simulink model "controllo_leggelin_e_quad"  (R2019b)
settings: Solver=FixedStepAuto  StartTime=0.0  StopTime=t_tot  FixedStep=dt  RelTol=1e-3
values from neighbouring files (symbols this model uses):
  A = [0 0 1 0; 0 0 0 1; 0 a_32  0 a_34; a_41 a_42 0 a_44]    [QuarterCarModel.m]
  B = [0; 0; 0; -kt/mu]    [QuarterCarModel.m]
  C = [0 -k/ms 0 -c_min/ms]    [QuarterCarModel.m]
  c_min = 800    [QuarterCarModel.m]
  er = 0.7    [QuarterCarModel.m]
  f_max = 3000    [QuarterCarModel.m]
  k = 27000    [QuarterCarModel.m]
  k0 = 38000    [QuarterCarModel.m]
  k_tilde = best_Ktilde    [QuarterCarModel.m]    (also in fun_lin.m = [x.k1 x.k2 x.k3 x.k4]; fun_lin_e_quad.m = [x.k1 0 x.k3 x.k4])
  kt = 300000    [QuarterCarModel.m]
  ms = 450    [QuarterCarModel.m]
  mu = 70    [QuarterCarModel.m]
  Px = best_elementsP    [QuarterCarModel.m]    (also in fun_lin_e_quad.m = [0 0 x.p13  x.p14; 0 0 0 0; x.p13 0 0  x.p34;  x.p14 0  x.p3; fun_quad.m = [x.p11 0 x.p13  x.p14; 0 0 0 0; x.p13 0 x.p33  x.p34;  x.p14)
  wr = 2*pi*v/lc    (= 7.85398163397)    [QuarterCarModel.m]
libraries: simulink x2
settings Model: Creator=Elia  LastModifiedBy=Elia

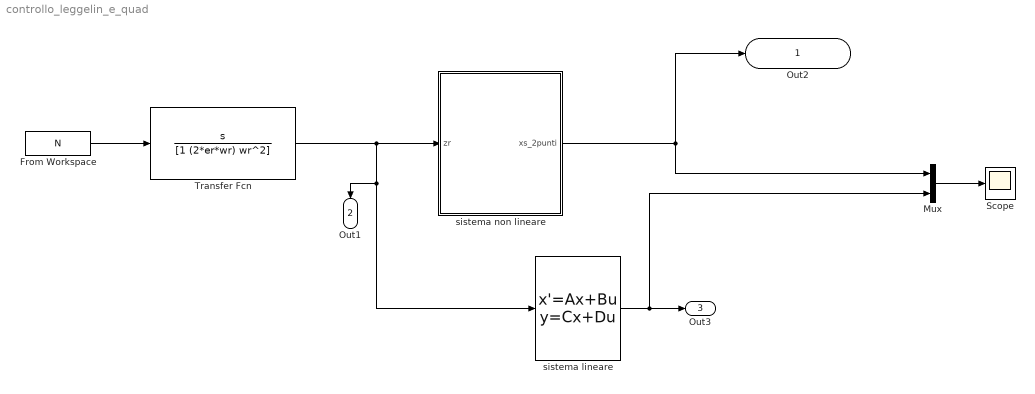
== system controllo_leggelin_e_quad ==
  From Workspace : FromWorkspace  VariableName=N  SampleTime=0
  Mux : Mux  Inputs=2
  Scope : Scope
  Transfer Fcn : TransferFcn  Numerator=[1 0]  Denominator=[1 (2*er*wr) wr^2]
  sistema lineare : StateSpace  A=A  B=B  C=C  D=0  InitialCondition=0
  sistema non lineare : Subsystem
  Out2 : Outport  SignalName=xs_2punti
  Out1 : Outport  Port=2  SignalName=zr
  Out3 : Outport  Port=3  SignalName=xs_2punti_lineare
  wires:
  sistema non lineare/1(xs_2punti) -> Mux/1, Out2/1
  From Workspace/1 -> Transfer Fcn/1
  Transfer Fcn/1 -> sistema non lineare/1(zr), sistema lineare/1, Out1/1
  sistema lineare/1 -> Mux/2, Out3/1
  Mux/1 -> Scope/1

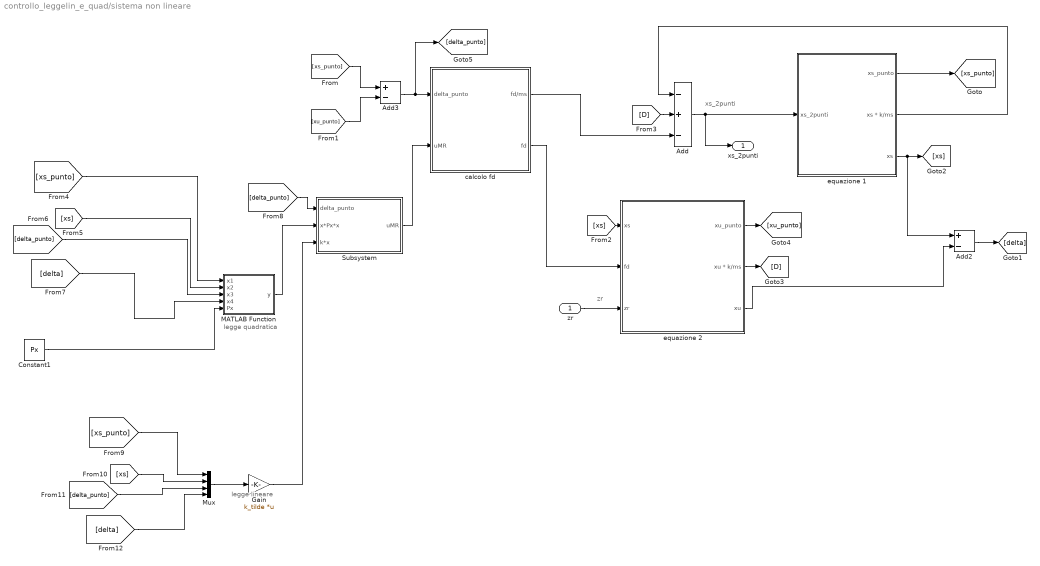
== system controllo_leggelin_e_quad/sistema non lineare ==
  note: legge quadratica
  note: xs_2punti
  note: zr
  note: legge lineare
  zr : Inport
  Add : Sum  Inputs=-+-
  Add2 : Sum  Inputs=+-
  Add3 : Sum  Inputs=+-
  Constant1 : Constant  Value=Px
  Gain : Gain  Gain=k_tilde  Multiplication=Matrix(K*u)
  MATLAB Function : MATLAB Function  TreatAsAtomicUnit=on
  Mux : Mux
  Subsystem : Subsystem
  calcolo fd : Subsystem
  equazione 1 : Subsystem
  equazione 2 : Subsystem
  xs_2punti : Outport
  wires:
  calcolo fd/2(fd) -> equazione 2/2(fd)
  equazione 1/3(xs) -> Add2/1, [xs]
  Add/1 -> xs_2punti/1, equazione 1/1(xs_2punti)
  equazione 1/1(xs_punto) -> [xs_punto]
  calcolo fd/1(fd/ms) -> Add/3
  [xs] -> equazione 2/1(xs)
  [D] -> Add/2
  equazione 1/2("xs * k/ms ") -> Add/1
  equazione 2/2("xu * k/ms ") -> [D]
  zr/1 -> equazione 2/3(zr)
  equazione 2/3(xu) -> Add2/2
  equazione 2/1(xu_punto) -> [xu_punto]
  [xu_punto] -> Add3/2
  [xs_punto] -> Add3/1
  Add3/1 -> [delta_punto], calcolo fd/1("delta_punto ")
  Add2/1 -> [delta]
  [delta_punto] -> Subsystem/1(delta_punto)
  MATLAB Function/1(y) -> Subsystem/2(x*Px*x)
  Constant1/1 -> MATLAB Function/5(Px)
  [xs_punto] -> MATLAB Function/1(x1)
  [xs] -> MATLAB Function/2(x2)
  [delta_punto] -> MATLAB Function/3(x3)
  [delta] -> MATLAB Function/4(x4)
  Subsystem/1(uMR) -> calcolo fd/2(uMR)
  [delta_punto] -> Mux/3
  [delta] -> Mux/4
  Mux/1 -> Gain/1
  [xs] -> Mux/2
  [xs_punto] -> Mux/1
  Gain/1 -> Subsystem/3(k*x)

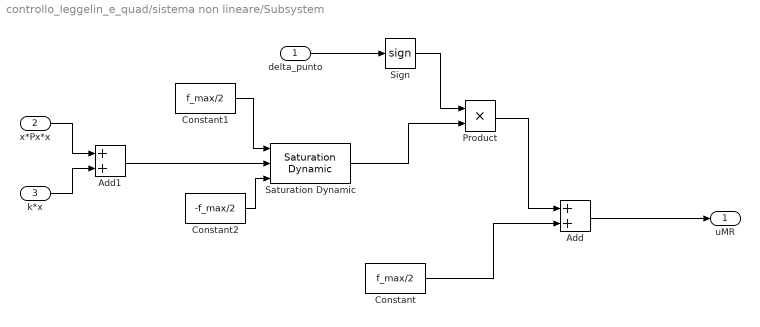
== system controllo_leggelin_e_quad/sistema non lineare/Subsystem ==
  delta_punto : Inport
  x*Px*x : Inport  Port=2
  k*x : Inport  Port=3
  Add : Sum
  Add1 : Sum
  Constant : Constant  Value=f_max/2
  Constant1 : Constant  Value=f_max/2
  Constant2 : Constant  Value=-f_max/2
  Product : Product
  Saturation Dynamic : simulink/Discontinuities/Saturation Dynamic  OutMin=[]  OutMax=[]  OutDataTypeStr=Inherit: Same as second input  OutDataType=fixdt(1, 16)  OutScaling=2^-10  DoSatur=off
  Sign : Signum
  uMR : Outport
  wires:
  Constant/1 -> Add/2
  Add/1 -> uMR/1
  delta_punto/1 -> Sign/1
  Saturation Dynamic/1 -> Product/2
  Sign/1 -> Product/1
  Product/1 -> Add/1
  Constant1/1 -> Saturation Dynamic/1
  Constant2/1 -> Saturation Dynamic/3
  x*Px*x/1 -> Add1/1
  k*x/1 -> Add1/2
  Add1/1 -> Saturation Dynamic/2

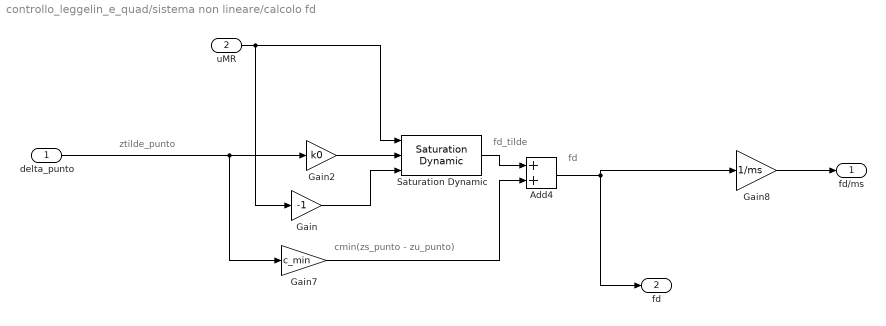
== system controllo_leggelin_e_quad/sistema non lineare/calcolo fd ==
  note: ztilde_punto
  note: cmin(zs_punto - zu_punto)
  note: fd
  note: fd_tilde
  "delta_punto " : Inport
  uMR : Inport  Port=2
  Add4 : Sum
  Gain : Gain  Gain=-1
  Gain2 : Gain  Gain=k0
  Gain7 : Gain  Gain=c_min
  Gain8 : Gain  Gain=1/ms
  Saturation Dynamic : simulink/Discontinuities/Saturation Dynamic  OutMin=[]  OutMax=[]  OutDataTypeStr=Inherit: Same as second input  OutDataType=fixdt(1, 16)  OutScaling=2^-10  DoSatur=off
  fd/ms : Outport
  fd : Outport  Port=2
  wires:
  "delta_punto "/1 -> Gain2/1, Gain7/1
  Gain2/1 -> Saturation Dynamic/2
  Add4/1 -> Gain8/1, fd/1
  Gain8/1 -> fd/ms/1
  Gain7/1 -> Add4/2
  Saturation Dynamic/1 -> Add4/1
  uMR/1 -> Gain/1, Saturation Dynamic/1
  Gain/1 -> Saturation Dynamic/3

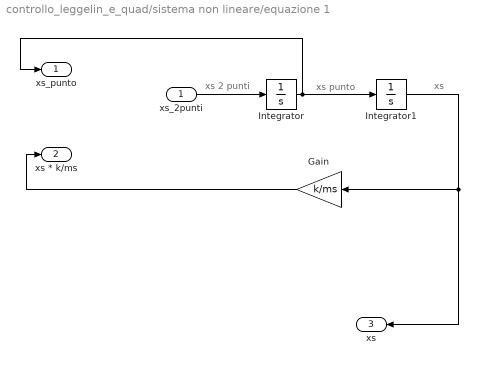
== system controllo_leggelin_e_quad/sistema non lineare/equazione 1 ==
  note: xs
  note: xs 2 punti
  note: xs punto
  xs_2punti : Inport
  Gain : Gain  Gain=k/ms
  Integrator : Integrator
  Integrator1 : Integrator
  xs_punto : Outport
  "xs * k/ms " : Outport  Port=2
  xs : Outport  Port=3
  wires:
  xs_2punti/1 -> Integrator/1
  Integrator/1 -> xs_punto/1, Integrator1/1
  Integrator1/1 -> xs/1, Gain/1
  Gain/1 -> "xs * k/ms "/1

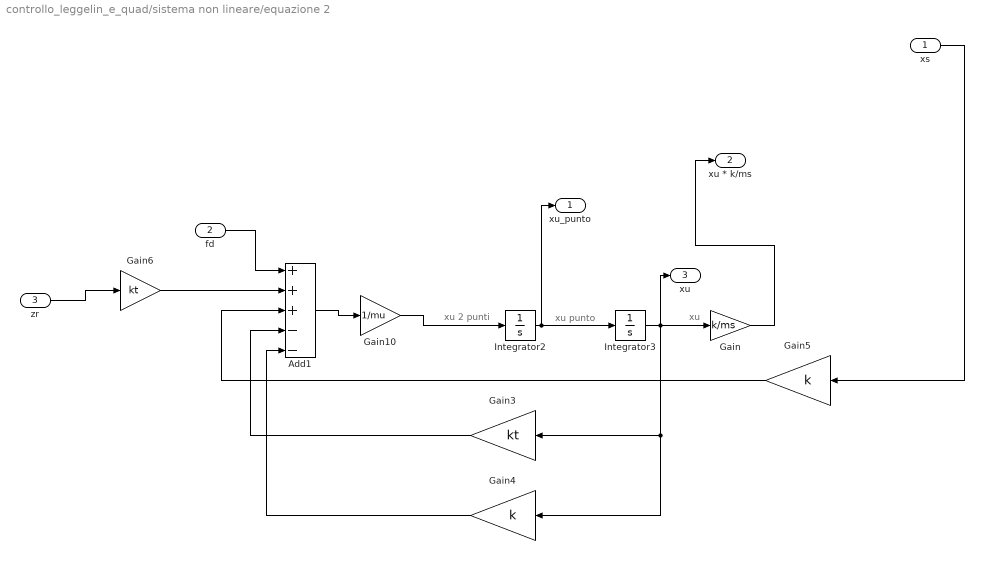
== system controllo_leggelin_e_quad/sistema non lineare/equazione 2 ==
  note: xu
  note: xu 2 punti
  note: xu punto
  xs : Inport
  fd : Inport  Port=2
  zr : Inport  Port=3
  Add1 : Sum  Inputs=+++--
  Gain : Gain  Gain=k/ms
  Gain10 : Gain  Gain=1/mu
  Gain3 : Gain  Gain=kt
  Gain4 : Gain  Gain=k
  Gain5 : Gain  Gain=k
  Gain6 : Gain  Gain=kt
  Integrator2 : Integrator
  Integrator3 : Integrator
  xu_punto : Outport
  "xu * k/ms " : Outport  Port=2
  xu : Outport  Port=3
  wires:
  Integrator2/1 -> xu_punto/1, Integrator3/1
  Integrator3/1 -> xu/1, Gain3/1, Gain4/1, Gain/1
  Gain6/1 -> Add1/2
  Add1/1 -> Gain10/1
  Gain10/1 -> Integrator2/1
  Gain3/1 -> Add1/4
  Gain5/1 -> Add1/3
  Gain4/1 -> Add1/5
  zr/1 -> Gain6/1
  xs/1 -> Gain5/1
  fd/1 -> Add1/1
  Gain/1 -> "xu * k/ms "/1

== matlab function controllo_leggelin_e_quad/sistema non lineare/MATLAB Function ==
  data: x1 input; x2 input; x3 input; x4 input; y output double size=[1 1]; Px input
function y = fcn(x1,x2,x3,x4,Px)
x = [x1;
     x2;
     x3;
     x4];
 
y = x.'*Px*x;
